simulink model "simulation_UCBF"  (R2022a)
settings: Solver=VariableStepAuto  StartTime=0.0  StopTime=simTime  RelTol=1e-3
values from neighbouring files (symbols this model uses):
  a = 0.1    [setup_UCBF.m]
  ContGainVec = [kp kd]    [setup_UCBF.m]
  Icm = 0.02    [setup_UCBF.m]
  m = 10    [setup_UCBF.m]
  params = [m,Icm,a]    [setup_UCBF.m]
  q0 = [0 0.5 1 0 0]    [setup_UCBF.m]
  qg = [x1d ;y1d]    [setup_UCBF.m]
settings Model: Creator=mirkomizzoni  LastModifiedBy=mirkomizzoni

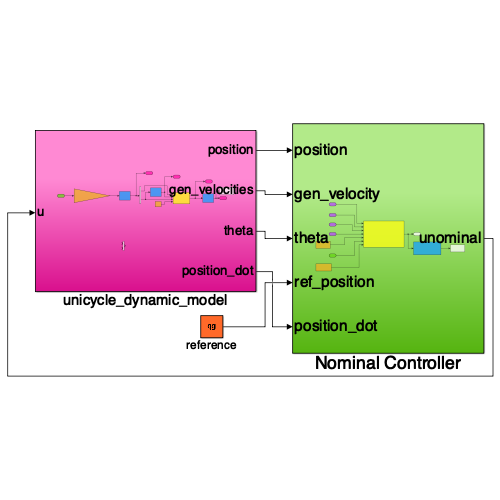
[thumbnail: Simulink's stored preview of the top-level diagram]
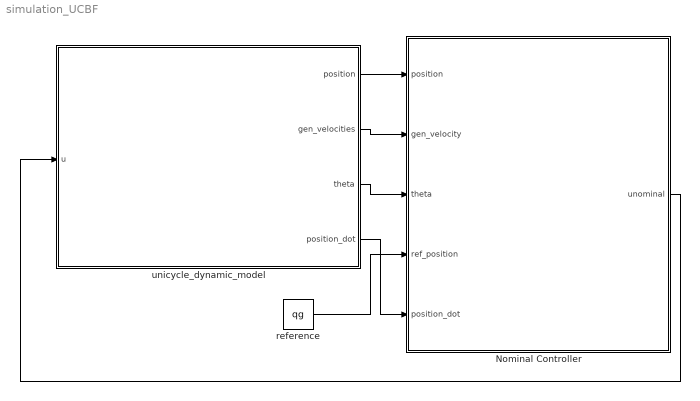
== system simulation_UCBF ==
  Nominal Controller : Subsystem
  reference : Constant  Value=qg
  unicycle_dynamic_model : Subsystem
  wires:
  reference/1 -> Nominal Controller/4(ref_position)
  unicycle_dynamic_model/2(gen_velocities) -> Nominal Controller/2(gen_velocity)
  unicycle_dynamic_model/3(theta) -> Nominal Controller/3(theta)
  unicycle_dynamic_model/1(position) -> Nominal Controller/1(position)
  unicycle_dynamic_model/4(position_dot) -> Nominal Controller/5(position_dot)
  Nominal Controller/1(unominal) -> unicycle_dynamic_model/1(u)

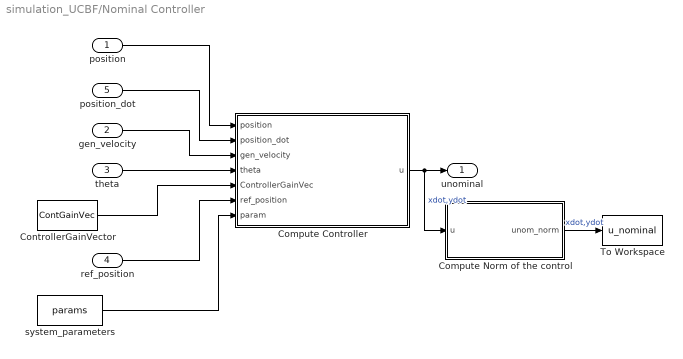
== system simulation_UCBF/Nominal Controller ==
  position : Inport
  gen_velocity : Inport  Port=2
  theta : Inport  Port=3
  ref_position : Inport  Port=4
  position_dot : Inport  Port=5
  Compute Controller : MATLAB Function  TreatAsAtomicUnit=on
  Compute Norm of the control : MATLAB Function  TreatAsAtomicUnit=on
  ControllerGainVector : Constant  Value=ContGainVec
  To Workspace : ToWorkspace  VariableName=u_nominal  SaveFormat=Timeseries  SampleTime=-1
  system_parameters : Constant  Value=params
  unominal : Outport
  wires:
  ref_position/1 -> Compute Controller/6(ref_position)
  ControllerGainVector/1 -> Compute Controller/5(ControllerGainVec)
  theta/1 -> Compute Controller/4(theta)
  position_dot/1 -> Compute Controller/2(position_dot)
  Compute Controller/1(u) -> unominal/1, Compute Norm of the control/1(u)  "xdot,ydot"
  position/1 -> Compute Controller/1(position)
  gen_velocity/1 -> Compute Controller/3(gen_velocity)
  system_parameters/1 -> Compute Controller/7(param)
  Compute Norm of the control/1(unom_norm) -> To Workspace/1  "xdot,ydot"

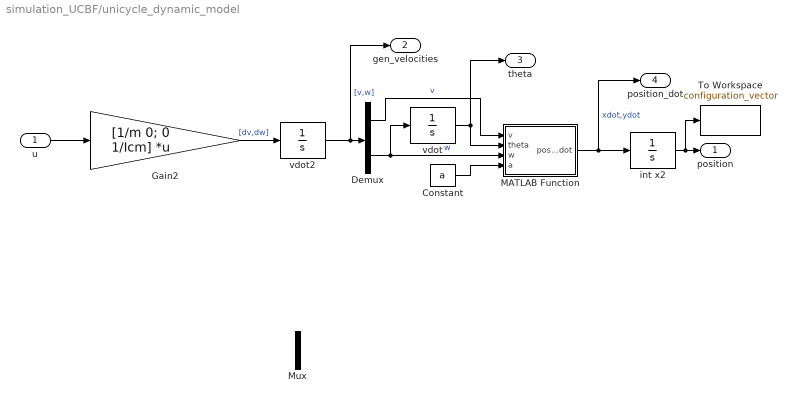
== system simulation_UCBF/unicycle_dynamic_model ==
  u : Inport
  Constant : Constant  Value=a
  Demux : Demux  Outputs=2
  Gain2 : Gain  Gain=[1/m 0; 0 1/Icm]  Multiplication=Matrix(K*u)
  MATLAB Function : MATLAB Function  TreatAsAtomicUnit=on
  Mux : Mux  Inputs=2
  To Workspace : ToWorkspace  VariableName=configuration_vector  SaveFormat=Timeseries  SampleTime=-1
  int x2 : Integrator  InitialCondition=[q0(1),q0(2)]
  vdot : Integrator  InitialCondition=q0(3)
  vdot2 : Integrator  InitialCondition=[q0(4);q0(5)]
  position : Outport
  gen_velocities : Outport  Port=2
  theta : Outport  Port=3
  position_dot : Outport  Port=4
  wires:
  vdot/1 -> theta/1, MATLAB Function/2(theta)
  Constant/1 -> MATLAB Function/4(a)
  Demux/2 -> vdot/1, MATLAB Function/3(w)  "w"
  vdot2/1 -> gen_velocities/1, Demux/1  "[v,w]"
  Gain2/1 -> vdot2/1  "[dv,dw]"
  int x2/1 -> To Workspace/1, position/1
  u/1 -> Gain2/1
  MATLAB Function/1(positiondot) -> position_dot/1, int x2/1  "xdot,ydot"
  Demux/1 -> MATLAB Function/1(v)  "v"

== matlab function simulation_UCBF/Nominal Controller/Compute Controller ==
  data: u output; position input; position_dot input; gen_velocity input; theta input; ControllerGainVec input; ref_position input; param input
function u = posdot(position,position_dot,gen_velocity,theta,ControllerGainVec,ref_position,param)
       v = gen_velocity(1);
       w = gen_velocity(2);
       m = param(1);
       Icm = param(2);
       a = param(3);
       g = [cos(theta)/m -a*sin(theta)/Icm ; sin(theta)/m a*cos(theta)/Icm];
       f = [-v*w*sin(theta)-w^2*a*cos(theta); v*w*cos(theta)-w^2*a*sin(theta)];
       kp = ControllerGainVec(1)*eye(2);
       kd = ControllerGainVec(2)*eye(2);
       vbar = kp*(ref_position-position)-kd*position_dot;
       % 2x2 2*1
       u = g^(-1)*(-f+vbar);
end

== matlab function simulation_UCBF/unicycle_dynamic_model/MATLAB Function ==
  data: v input; positiondot output; theta input; w input; a input
function positiondot = posdot(v,theta,w,a)
        dx = v*cos(theta)-w*a*sin(theta);
        dy = v*sin(theta)+w*a*cos(theta);
        positiondot = [dx;dy];
end

== matlab function simulation_UCBF/Nominal Controller/Compute Norm of the control ==
  data: unom_norm output; u input
function unom_norm = norm_control(u)
    unom_norm = norm(u);
end
